simulink model "ModelMarco_Full"  (R2018a)
settings: Solver=FixedStepAuto  StartTime=0  StopTime=1382400  FixedStep=5  RelTol=1e-1
undefined symbols (not defined in the file or in its folder): magnitude
libraries: simulink x2
(part 2 of 2)

== system ModelMarco_Full/RoofStrategy ==
  Tset_vent : Inport
  RHset_vent : Inport  Port=2
  T_air : Inport  Port=3
  RH : Inport  Port=4
  RH_out : Inport  Port=5
  I : Inport  Port=6
  Constant : Constant  Value=0
  Gain : Gain
  Gain1 : Gain  Gain=0
  MATLAB Function : MATLAB Function  TreatAsAtomicUnit=on
  MATLAB Function1 : MATLAB Function  TreatAsAtomicUnit=on
  Saturation : Saturate  UpperLimit=1  LowerLimit=0
  Scope : Scope
  Sum : Sum  Inputs=|++
  day/night : Switch  Criteria=u2 > Threshold  Threshold=20
  Uroof : Outport
  wires:
  T_air/1 -> MATLAB Function/1(T_air)
  Tset_vent/1 -> MATLAB Function/2(Tset)
  RH/1 -> MATLAB Function1/1(RH_air)
  RH_out/1 -> MATLAB Function1/2(RH_out)
  RHset_vent/1 -> MATLAB Function1/3(RH_set)
  MATLAB Function/1(y) -> Gain/1
  MATLAB Function1/1(y) -> Gain1/1
  Gain/1 -> Sum/1
  Gain1/1 -> Sum/2
  Sum/1 -> Saturation/1
  I/1 -> day/night/2
  day/night/1 -> Scope/1, Uroof/1
  Saturation/1 -> day/night/1
  Constant/1 -> day/night/3

== system ModelMarco_Full/Scr(Scr->Covin) ==
  A_floor : Inport
  T_scr : Inport  Port=2
  T_covin : Inport  Port=3
  U_Thrscr : Inport  Port=4
  " Stefan-Boltzmann constant" : Constant  Value=5.67e-8
  " epsilon_cov" : Constant  Value=0.9
  " epsilon_scr" : Constant  Value=0.44
  Bias : Bias  Bias=273.15
  Bias1 : Bias  Bias=273.15
  Fcn : Fcn  Expr=u^4
  Fcn1 : Fcn  Expr=u^4
  Product : Product  Inputs=6
  Sum : Sum  Inputs=|+-
  R_FIR_scr->covin : Outport
  wires:
  A_floor/1 -> Product/1  "A_floor"
  T_scr/1 -> Bias/1
  T_covin/1 -> Bias1/1
  Bias/1 -> Fcn/1
  Bias1/1 -> Fcn1/1
  Fcn/1 -> Sum/1
  Fcn1/1 -> Sum/2
  Sum/1 -> Product/3
  Product/1 -> R_FIR_scr->covin/1
  " Stefan-Boltzmann constant"/1 -> Product/4
  " epsilon_cov"/1 -> Product/2
  U_Thrscr/1 -> Product/5  "F"
  " epsilon_scr"/1 -> Product/6

== system ModelMarco_Full/Scr(Scr->sky) ==
  A_floor : Inport
  T_scr : Inport  Port=2
  T_sky : Inport  Port=3
  U_Thrscr : Inport  Port=4
  " Stefan-Boltzmann constant" : Constant  Value=5.67e-8
  " epsilon_scr" : Constant  Value=0.44
  " epsilon_sky" : Constant
  Bias : Bias  Bias=273.15
  Bias1 : Bias  Bias=273.15
  Fcn : Fcn  Expr=u^4
  Fcn1 : Fcn  Expr=u^4
  Product : Product  Inputs=6
  Sum : Sum  Inputs=|+-
  tau_cov : Gain  Gain=0
  R_FIR_scr->sky : Outport
  wires:
  A_floor/1 -> Product/1  "A_floor"
  T_scr/1 -> Bias/1
  T_sky/1 -> Bias1/1
  Bias/1 -> Fcn/1
  Bias1/1 -> Fcn1/1
  Fcn/1 -> Sum/1
  Fcn1/1 -> Sum/2
  Sum/1 -> Product/3
  Product/1 -> R_FIR_scr->sky/1
  " Stefan-Boltzmann constant"/1 -> Product/4
  " epsilon_sky"/1 -> Product/2
  U_Thrscr/1 -> tau_cov/1
  tau_cov/1 -> Product/5  "F"
  " epsilon_scr"/1 -> Product/6

== system ModelMarco_Full/Scr(can->scr) ==
  A_floor : Inport
  T_can : Inport  Port=2
  T_scr : Inport  Port=3
  U_Thrscr : Inport  Port=4
  LAI : Inport  Port=5
  " Stefan-Boltzmann constant" : Constant  Value=5.67e-8
  " epsilon_can" : Constant
  " epsilon_scr" : Constant  Value=0.44
  Bias : Bias  Bias=273.15
  Bias1 : Bias  Bias=273.15
  Fcn : Fcn  Expr=u^4
  Fcn1 : Fcn  Expr=u^4
  Fcn2 : Fcn  Expr=1-exp(-0.94*u)
  Product : Product  Inputs=6
  Product1 : Product
  Sum : Sum  Inputs=|+-
  R_FIR_can->scr : Outport
  wires:
  T_can/1 -> Bias/1
  T_scr/1 -> Bias1/1
  Bias/1 -> Fcn/1
  Bias1/1 -> Fcn1/1
  Fcn/1 -> Sum/1
  Fcn1/1 -> Sum/2
  Sum/1 -> Product/3
  Product/1 -> R_FIR_can->scr/1
  " Stefan-Boltzmann constant"/1 -> Product/4
  " epsilon_scr"/1 -> Product/2
  U_Thrscr/1 -> Product/5  "F"
  " epsilon_can"/1 -> Product/6
  LAI/1 -> Fcn2/1
  Product1/1 -> Product/1
  A_floor/1 -> Product1/2  "A_floor"
  Fcn2/1 -> Product1/1

== system ModelMarco_Full/Scr(floor->scr) ==
  A_floor : Inport
  T_floor : Inport  Port=2
  T_scr : Inport  Port=3
  U_Thrscr : Inport  Port=4
  LAI : Inport  Port=5
  " Stefan-Boltzmann constant" : Constant  Value=5.67e-8
  " epsilon_floor" : Constant
  " epsilon_scr" : Constant  Value=0.44
  Bias : Bias  Bias=273.15
  Bias1 : Bias  Bias=273.15
  Fcn : Fcn  Expr=u^4
  Fcn1 : Fcn  Expr=u^4
  Fcn2 : Fcn  Expr=exp(-0.94*u)
  Product : Product  Inputs=6
  Product1 : Product
  Sum : Sum  Inputs=|+-
  R_FIR_floor->scr : Outport
  wires:
  T_floor/1 -> Bias/1
  T_scr/1 -> Bias1/1
  Bias/1 -> Fcn/1
  Bias1/1 -> Fcn1/1
  Fcn/1 -> Sum/1
  Fcn1/1 -> Sum/2
  Sum/1 -> Product/3
  Product/1 -> R_FIR_floor->scr/1
  " Stefan-Boltzmann constant"/1 -> Product/4
  " epsilon_scr"/1 -> Product/2
  " epsilon_floor"/1 -> Product/6
  A_floor/1 -> Product/1
  LAI/1 -> Fcn2/1
  Product1/1 -> Product/5
  Fcn2/1 -> Product1/1
  U_Thrscr/1 -> Product1/2

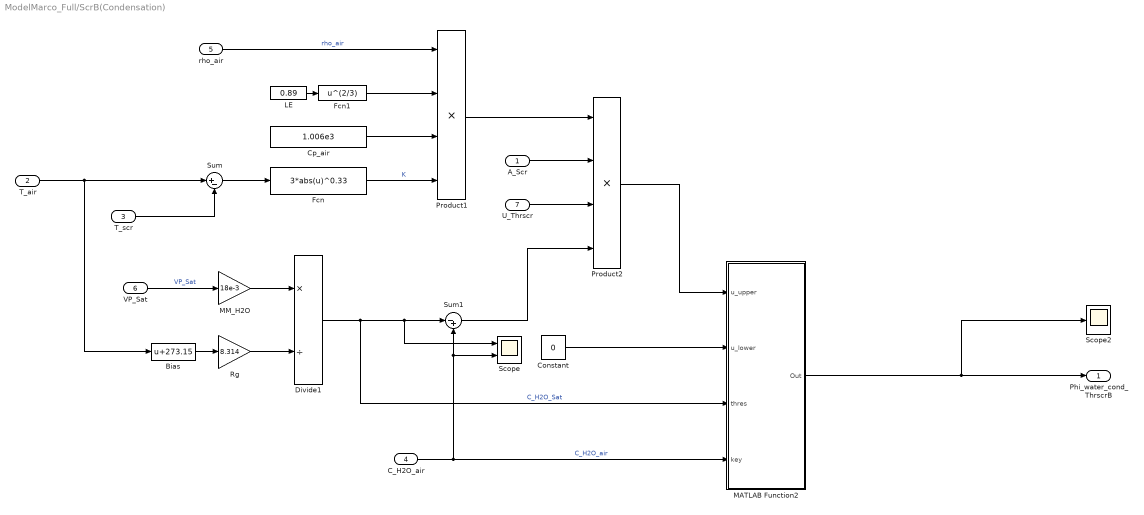
== system ModelMarco_Full/ScrB(Condensation) ==
  A_Scr : Inport
  T_air : Inport  Port=2
  T_scr : Inport  Port=3
  C_H2O_air : Inport  Port=4
  rho_air : Inport  Port=5
  VP_Sat : Inport  Port=6
  U_Thrscr : Inport  Port=7
  Bias : Bias  Bias=273.15
  Constant : Constant  Value=0
  Cp_air : Constant  Value=1.006e3
  Divide1 : Product  Inputs=*/
  Fcn : Fcn  Expr=3*abs(u)^0.33
  Fcn1 : Fcn  Expr=u^(2/3)
  LE : Constant  Value=0.89
  MATLAB Function2 : MATLAB Function  TreatAsAtomicUnit=on
  MM_H2O : Gain  Gain=18e-3
  Product1 : Product  Inputs=4
  Product2 : Product  Inputs=4
  Rg : Gain  Gain=8.314
  Scope : Scope  NumInputPorts=2
  Scope2 : Scope
  Sum : Sum  Inputs=|+-
  Sum1 : Sum  Inputs=|-+
  Phi_water_cond_ThrscrB : Outport
  wires:
  T_air/1 -> Sum/1, Bias/1
  T_scr/1 -> Sum/2
  Sum/1 -> Fcn/1
  Bias/1 -> Rg/1
  Rg/1 -> Divide1/2
  rho_air/1 -> Product1/1  "rho_air"
  LE/1 -> Fcn1/1
  Fcn1/1 -> Product1/2
  Cp_air/1 -> Product1/3
  Fcn/1 -> Product1/4  "K"
  VP_Sat/1 -> MM_H2O/1  "VP_Sat"
  MM_H2O/1 -> Divide1/1
  Divide1/1 -> MATLAB Function2/3(thres), Scope/1, Sum1/1  "C_H2O_Sat"
  C_H2O_air/1 -> Scope/2, Sum1/2, MATLAB Function2/4(key)  "C_H2O_air"
  Product1/1 -> Product2/1
  A_Scr/1 -> Product2/2
  Constant/1 -> MATLAB Function2/2(u_lower)
  Product2/1 -> MATLAB Function2/1(u_upper)
  MATLAB Function2/1(Out) -> Scope2/1, Phi_water_cond_ThrscrB/1
  Sum1/1 -> Product2/4
  U_Thrscr/1 -> Product2/3

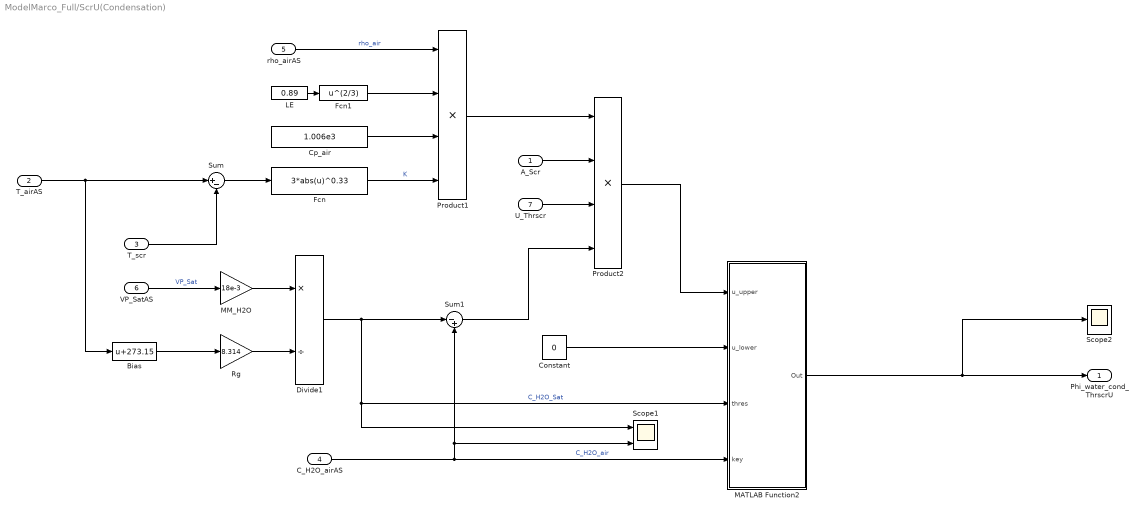
== system ModelMarco_Full/ScrU(Condensation) ==
  A_Scr : Inport
  T_airAS : Inport  Port=2
  T_scr : Inport  Port=3
  C_H2O_airAS : Inport  Port=4
  rho_airAS : Inport  Port=5
  VP_SatAS : Inport  Port=6
  U_Thrscr : Inport  Port=7
  Bias : Bias  Bias=273.15
  Constant : Constant  Value=0
  Cp_air : Constant  Value=1.006e3
  Divide1 : Product  Inputs=*/
  Fcn : Fcn  Expr=3*abs(u)^0.33
  Fcn1 : Fcn  Expr=u^(2/3)
  LE : Constant  Value=0.89
  MATLAB Function2 : MATLAB Function  TreatAsAtomicUnit=on
  MM_H2O : Gain  Gain=18e-3
  Product1 : Product  Inputs=4
  Product2 : Product  Inputs=4
  Rg : Gain  Gain=8.314
  Scope1 : Scope  NumInputPorts=2
  Scope2 : Scope
  Sum : Sum  Inputs=|+-
  Sum1 : Sum  Inputs=|-+
  Phi_water_cond_ThrscrU : Outport
  wires:
  T_airAS/1 -> Sum/1, Bias/1
  T_scr/1 -> Sum/2
  Sum/1 -> Fcn/1
  Bias/1 -> Rg/1
  Rg/1 -> Divide1/2
  rho_airAS/1 -> Product1/1  "rho_air"
  LE/1 -> Fcn1/1
  Fcn1/1 -> Product1/2
  Cp_air/1 -> Product1/3
  Fcn/1 -> Product1/4  "K"
  VP_SatAS/1 -> MM_H2O/1  "VP_Sat"
  MM_H2O/1 -> Divide1/1
  Divide1/1 -> Scope1/1, MATLAB Function2/3(thres), Sum1/1  "C_H2O_Sat"
  C_H2O_airAS/1 -> Scope1/2, Sum1/2, MATLAB Function2/4(key)  "C_H2O_air"
  Product1/1 -> Product2/1
  A_Scr/1 -> Product2/2
  Constant/1 -> MATLAB Function2/2(u_lower)
  Product2/1 -> MATLAB Function2/1(u_upper)
  MATLAB Function2/1(Out) -> Scope2/1, Phi_water_cond_ThrscrU/1
  Sum1/1 -> Product2/4
  U_Thrscr/1 -> Product2/3

== system ModelMarco_Full/Screen(Air->airAS) ==
  Phi_airASair : Inport
  T_air : Inport  Port=2
  T_airAS : Inport  Port=3
  Cp_air : Constant  Value=1.006e3
  Product : Product  Inputs=3
  Sum : Sum  Inputs=|+-
  Q_air->airAS : Outport
  wires:
  T_air/1 -> Sum/1
  T_airAS/1 -> Sum/2
  Sum/1 -> Product/3
  Cp_air/1 -> Product/1
  Phi_airASair/1 -> Product/2
  Product/1 -> Q_air->airAS/1

== system ModelMarco_Full/Screen(AirAs->scr) ==
  A_floor : Inport
  T_scr : Inport  Port=2
  T_airAS : Inport  Port=3
  U_Thrscr : Inport  Port=4
  Fcn : Fcn  Expr=1.7*abs(u)^0.33
  Product : Product  Inputs=3
  Product1 : Product
  Sum : Sum  Inputs=|+-
  Q_airAS->scr : Outport
  wires:
  T_airAS/1 -> Sum/1
  T_scr/1 -> Sum/2
  Sum/1 -> Fcn/1, Product/2
  A_floor/1 -> Product/1
  Product1/1 -> Product/3  "K"
  Fcn/1 -> Product1/1
  U_Thrscr/1 -> Product1/2
  Product/1 -> Q_airAS->scr/1

== system ModelMarco_Full/Screen(scr->air) ==
  A_floor : Inport
  T_air : Inport  Port=2
  T_scr : Inport  Port=3
  U_Thrscr : Inport  Port=4
  Fcn : Fcn  Expr=1.7*abs(u)^0.33
  Product : Product  Inputs=3
  Product1 : Product
  Sum : Sum  Inputs=|+-
  Q_scrair : Outport
  wires:
  T_scr/1 -> Sum/1
  T_air/1 -> Sum/2
  Sum/1 -> Fcn/1, Product/2
  A_floor/1 -> Product/1
  Product1/1 -> Product/3  "K"
  Fcn/1 -> Product1/1
  U_Thrscr/1 -> Product1/2
  Product/1 -> Q_scrair/1

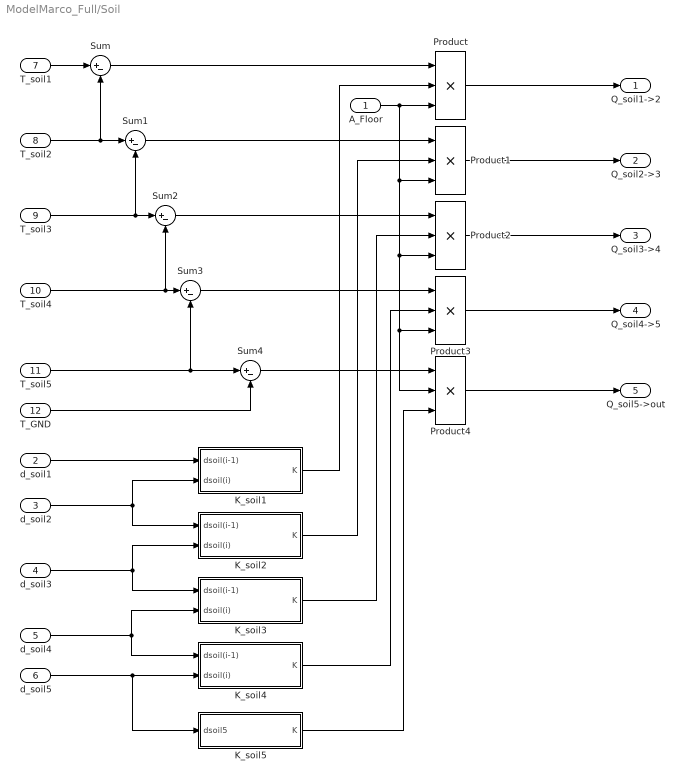
== system ModelMarco_Full/Soil ==
  A_Floor : Inport
  d_soil1 : Inport  Port=2
  d_soil2 : Inport  Port=3
  d_soil3 : Inport  Port=4
  d_soil4 : Inport  Port=5
  d_soil5 : Inport  Port=6
  T_soil1 : Inport  Port=7
  T_soil2 : Inport  Port=8
  T_soil3 : Inport  Port=9
  T_soil4 : Inport  Port=10
  T_soil5 : Inport  Port=11
  T_GND : Inport  Port=12
  K_soil1 : Subsystem
  K_soil2 : Subsystem
  K_soil3 : Subsystem
  K_soil4 : Subsystem
  K_soil5 : Subsystem
  Product{,1..4} (5 alike) : Product  Inputs=3
  Sum{,1..4} (5 alike) : Sum  Inputs=|+-
  Q_soil1->2 : Outport
  Q_soil2->3 : Outport  Port=2
  Q_soil3->4 : Outport  Port=3
  Q_soil4->5 : Outport  Port=4
  Q_soil5->out : Outport  Port=5
  wires:
  d_soil2/1 -> K_soil1/2(dsoil(i)), K_soil2/1(dsoil(i-1))
  d_soil1/1 -> K_soil1/1(dsoil(i-1))
  d_soil3/1 -> K_soil3/1(dsoil(i-1)), K_soil2/2(dsoil(i))
  d_soil4/1 -> K_soil3/2(dsoil(i)), K_soil4/1(dsoil(i-1))
  d_soil5/1 -> K_soil5/1(dsoil5), K_soil4/2(dsoil(i))
  T_soil1/1 -> Sum/1
  T_soil2/1 -> Sum/2, Sum1/1
  Sum/1 -> Product/1
  K_soil1/1(K) -> Product/2
  A_Floor/1 -> Product2/3, Product4/2, Product3/3, Product1/3, Product/3
  Product/1 -> Q_soil1->2/1
  Sum1/1 -> Product1/1
  K_soil2/1(K) -> Product1/2
  Product1/1 -> Q_soil2->3/1
  T_soil3/1 -> Sum2/1, Sum1/2
  Sum2/1 -> Product2/1
  T_soil4/1 -> Sum3/1, Sum2/2
  Sum3/1 -> Product3/1
  K_soil3/1(K) -> Product2/2
  T_soil5/1 -> Sum3/2, Sum4/1
  K_soil4/1(K) -> Product3/2
  Product2/1 -> Q_soil3->4/1
  Product3/1 -> Q_soil4->5/1
  T_GND/1 -> Sum4/2
  Sum4/1 -> Product4/1
  K_soil5/1(K) -> Product4/3
  Product4/1 -> Q_soil5->out/1

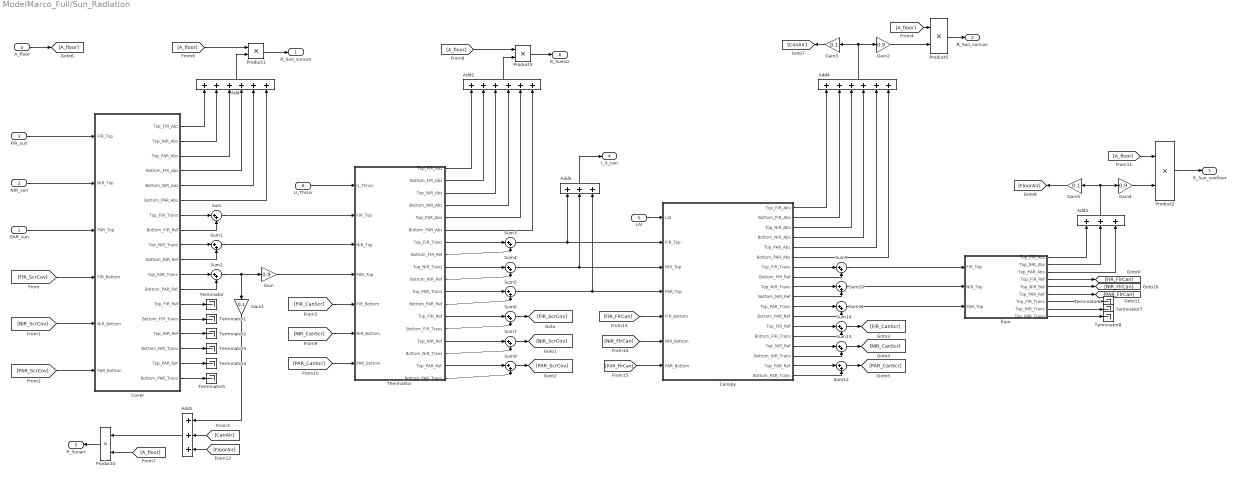
== system ModelMarco_Full/Sun_Radiation ==
  PAR_sun : Inport
  NIR_sun : Inport  Port=2
  FIR_sun : Inport  Port=3
  A_floor : Inport  Port=4
  LAI : Inport  Port=5
  U_Thrscr : Inport  Port=6
  Add : Sum  Inputs=++++++
  Add1 : Sum  Inputs=+++
  Add2 : Sum  Inputs=++++++
  Add3 : Sum  Inputs=+++
  Add4 : Sum  Inputs=++++++
  Add5 : Sum  Inputs=+++
  Canopy : Subsystem
  Cover : Subsystem
  Gain : Gain  Gain=0.9
  Gain1 : Gain  Gain=0.1
  Gain2 : Gain  Gain=0.9
  Gain3 : Gain  Gain=0.1
  Gain4 : Gain  Gain=0.9
  Gain5 : Gain  Gain=0.1
  Product{1..5} (5 alike) : Product
  Sum{,1..14} (15 alike) : Sum  Inputs=|++
  Terminator{,1..8} (9 alike) : Terminator
  ThermalScr : Subsystem
  floor : Subsystem
  R_Sun_suncov : Outport
  R_Sun_suncan : Outport  Port=2
  R_Sun_sunfloor : Outport  Port=3
  I_A_can : Outport  Port=4
  R_Sunair : Outport  Port=5
  "R_Sunscr " : Outport  Port=6
  wires:
  [FIR_ScrCov] -> Cover/4(FIR_Bottom)
  [NIR_ScrCov] -> Cover/5(NIR_Bottom)
  [PAR_ScrCov] -> Cover/6(PAR_Bottom)
  Product2/1 -> R_Sun_sunfloor/1
  [FIR_FlrCan] -> Canopy/5(FIR_Bottom)
  [NIR_FlrCan] -> Canopy/6(NIR_Bottom)
  [PAR_FlrCan] -> Canopy/7(PAR_Bottom)
  PAR_sun/1 -> Cover/3(PAR_Top)
  A_floor/1 -> [A_floor]
  LAI/1 -> Canopy/1(LAI)
  Cover/1(Top_FIR_Abs) -> Add/1
  Cover/2(Top_NIR_Abs) -> Add/2
  Cover/3(Top_PAR_Abs) -> Add/3
  Cover/4(Bottom_FIR_Abs) -> Add/4
  Cover/5(Bottom_NIR_Abs) -> Add/5
  Cover/6(Bottom_PAR_Abs) -> Add/6
  [A_floor] -> Product1/1
  Add/1 -> Product1/2
  Product1/1 -> R_Sun_suncov/1
  Cover/7(Top_FIR_Trans) -> Sum/1
  Cover/8(Bottom_FIR_Ref) -> Sum/2
  Cover/9(Top_NIR_Trans) -> Sum1/1
  Cover/10(Bottom_NIR_Ref) -> Sum1/2
  Cover/11(Top_PAR_Trans) -> Sum2/1
  Cover/12(Bottom_PAR_Ref) -> Sum2/2
  Sum/1 -> ThermalScr/2(FIR_Top)
  Sum1/1 -> ThermalScr/3(NIR_Top)
  Cover/13(Top_FIR_Ref) -> Terminator/1
  Cover/14(Bottom_FIR_Trans) -> Terminator1/1
  Cover/15(Top_NIR_Ref) -> Terminator2/1
  Cover/16(Bottom_NIR_Trans) -> Terminator3/1
  Cover/17(Top_PAR_Ref) -> Terminator4/1
  Cover/18(Bottom_PAR_Trans) -> Terminator5/1
  U_Thrscr/1 -> ThermalScr/1(U_Thrscr)
  NIR_sun/1 -> Cover/2(NIR_Top)
  FIR_sun/1 -> Cover/1(FIR_Top)
  Gain/1 -> ThermalScr/4(PAR_Top)
  Sum2/1 -> Gain1/1, Gain/1
  Gain1/1 -> Add1/1
  Add1/1 -> Product4/1
  [A_floor] -> Product4/2
  Product4/1 -> R_Sunair/1
  ThermalScr/1(Top_FIR_Abs) -> Add2/1
  ThermalScr/2(Bottom_FIR_Abs) -> Add2/2
  ThermalScr/3(Top_NIR_Abs) -> Add2/3
  ThermalScr/4(Bottom_NIR_Abs) -> Add2/4
  ThermalScr/5(Top_PAR_Abs) -> Add2/5
  ThermalScr/6(Bottom_PAR_Abs) -> Add2/6
  [A_floor] -> Product3/1
  Add2/1 -> Product3/2
  Product3/1 -> "R_Sunscr "/1
  ThermalScr/7(Top_FIR_Trans) -> Sum3/1
  ThermalScr/8(Bottom_FIR_Ref) -> Sum3/2
  ThermalScr/9(Top_NIR_Trans) -> Sum4/1
  ThermalScr/10(Bottom_NIR_Ref) -> Sum4/2
  ThermalScr/11(Top_PAR_Trans) -> Sum5/1
  ThermalScr/12(Bottom_PAR_Ref) -> Sum5/2
  Sum3/1 -> Add5/1, Canopy/2(FIR_Top)
  Sum4/1 -> Add5/2, Canopy/3(NIR_Top)
  Sum5/1 -> Add5/3, Canopy/4(PAR_Top)
  Sum6/1 -> [FIR_ScrCov]
  ThermalScr/13(Top_FIR_Ref) -> Sum6/1
  ThermalScr/14(Bottom_FIR_Trans) -> Sum6/2
  ThermalScr/15(Top_NIR_Ref) -> Sum7/1
  ThermalScr/16(Bottom_NIR_Trans) -> Sum7/2
  Sum7/1 -> [NIR_ScrCov]
  ThermalScr/17(Top_PAR_Ref) -> Sum8/1
  ThermalScr/18(Bottom_PAR_Trans) -> Sum8/2
  Sum8/1 -> [PAR_ScrCov]
  Canopy/1(Top_FIR_Abs) -> Add4/1
  Canopy/2(Bottom_FIR_Abs) -> Add4/2
  Canopy/3(Top_NIR_Abs) -> Add4/3
  Canopy/4(Bottom_NIR_Abs) -> Add4/4
  Canopy/5(Top_PAR_Abs) -> Add4/5
  Canopy/6(Bottom_PAR_Abs) -> Add4/6
  Add4/1 -> Gain2/1, Gain3/1
  Gain3/1 -> [CanAir]
  [CanAir] -> Add1/2
  Product5/1 -> R_Sun_suncan/1
  [A_floor] -> Product5/1
  Gain2/1 -> Product5/2
  Canopy/7(Top_FIR_Trans) -> Sum9/1
  Canopy/9(Top_NIR_Trans) -> Sum10/1
  Canopy/11(Top_PAR_Trans) -> Sum11/1
  Canopy/8(Bottom_FIR_Ref) -> Sum9/2
  Canopy/10(Bottom_NIR_Ref) -> Sum10/2
  Canopy/12(Bottom_PAR_Ref) -> Sum11/2
  Sum9/1 -> floor/1(FIR_Top)
  Sum10/1 -> floor/2(NIR_Top)
  Sum11/1 -> floor/3(PAR_Top)
  Canopy/13(Top_FIR_Ref) -> Sum14/1
  Canopy/14(Bottom_FIR_Trans) -> Sum14/2
  Canopy/15(Top_NIR_Ref) -> Sum13/1
  Canopy/16(Bottom_NIR_Trans) -> Sum13/2
  Canopy/17(Top_PAR_Ref) -> Sum12/1
  Canopy/18(Bottom_PAR_Trans) -> Sum12/2
  Add5/1 -> I_A_can/1
  Sum14/1 -> [FIR_CanScr]
  Sum13/1 -> [NIR_CanScr]
  Sum12/1 -> [PAR_CanScr]
  [FIR_CanScr] -> ThermalScr/5(FIR_Bottom)
  [NIR_CanScr] -> ThermalScr/6(NIR_Bottom)
  [PAR_CanScr] -> ThermalScr/7(PAR_Bottom)
  floor/1(Top_FIR_Abs) -> Add3/1
  floor/2(Top_NIR_Abs) -> Add3/2
  floor/3(Top_PAR_Abs) -> Add3/3
  Add3/1 -> Gain4/1, Gain5/1
  Gain4/1 -> Product2/2
  [A_floor] -> Product2/1
  Gain5/1 -> [FloorAir]
  [FloorAir] -> Add1/3
  floor/9(Top_PAR_Trans) -> Terminator8/1
  floor/8(Top_NIR_Trans) -> Terminator7/1
  floor/7(Top_FIR_Trans) -> Terminator6/1
  floor/4(Top_FIR_Ref) -> [FIR_FlrCan]
  floor/5(Top_NIR_Ref) -> [NIR_FlrCan]
  floor/6(Top_PAR_Ref) -> [PAR_FlrCan]

== system ModelMarco_Full/Vent ==
  rho_airAS : Inport
  Phi_roofvent : Inport  Port=2
  T_airAS : Inport  Port=3
  Tout : Inport  Port=4
  Cp_air : Constant  Value=1.006e3
  Product : Product  Inputs=4
  Sum : Sum  Inputs=|+-
  Q_roofvent : Outport
  wires:
  T_airAS/1 -> Sum/1
  Tout/1 -> Sum/2
  Sum/1 -> Product/4
  rho_airAS/1 -> Product/2
  Phi_roofvent/1 -> Product/3
  Cp_air/1 -> Product/1
  Product/1 -> Q_roofvent/1

== system ModelMarco_Full/Wall(air->out) ==
  Tout : Inport
  Tair : Inport  Port=2
  U : Inport  Port=3
  A_wall : Inport  Port=4
  Gain : Gain
  Product : Product  Inputs=3
  Sum : Sum  Inputs=|+-
  Q_air->out : Outport
  wires:
  Tair/1 -> Sum/1
  Tout/1 -> Sum/2
  Sum/1 -> Product/3
  U/1 -> Product/2
  A_wall/1 -> Product/1
  Gain/1 -> Q_air->out/1
  Product/1 -> Gain/1

== system ModelMarco_Full/Water_flow(ThrScr) ==
  Phi_leakage : Inport
  C_H2O_Air : Inport  Port=2
  C_H2O_AirAs : Inport  Port=3
  Product : Product
  Sum : Sum  Inputs=|+-
  Phi_water_ThrScr : Outport
  wires:
  C_H2O_Air/1 -> Sum/1
  C_H2O_AirAs/1 -> Sum/2
  Phi_leakage/1 -> Product/1
  Sum/1 -> Product/2
  Product/1 -> Phi_water_ThrScr/1

== system ModelMarco_Full/Water_flow(leakage) ==
  Phi_leakage : Inport
  C_H2O_in : Inport  Port=2
  C_H2O_out : Inport  Port=3
  Product : Product
  Sum : Sum  Inputs=|+-
  Phi_water_leak : Outport
  wires:
  C_H2O_in/1 -> Sum/1
  C_H2O_out/1 -> Sum/2
  Phi_leakage/1 -> Product/1
  Sum/1 -> Product/2
  Product/1 -> Phi_water_leak/1

== system ModelMarco_Full/Water_flow(roofvent) ==
  Phi_roofvent : Inport
  C_H2O_AS : Inport  Port=2
  C_H2O_out : Inport  Port=3
  Product : Product
  Sum : Sum  Inputs=|+-
  Phi_water_roofvent : Outport
  wires:
  C_H2O_AS/1 -> Sum/1
  C_H2O_out/1 -> Sum/2
  Phi_roofvent/1 -> Product/1
  Sum/1 -> Product/2
  Product/1 -> Phi_water_roofvent/1

== system ModelMarco_Full/Plants(transpiration)/Boundary Resistance ==
  note: Different Paper give different suggestion, not senstive
  T_can : Inport
  T_air : Inport  Port=2
  Abs : Abs
  Divide1 : Product  Inputs=**/
  Fcn : Fcn  Expr=u^(2/3)
  Fcn1 : Fcn  Expr=u^(1/4)
  Gain : Gain  Gain=1147
  Gain1 : Gain  Gain=207
  Le : Constant  Value=0.89
  Lf : Constant  Value=0.055
  Manual Switch : ManualSwitch  CurrentSetting=0
  Math Function : Math  Operator=magnitude^2  SaturateOnIntegerOverflow=on
  Product2 : Product
  Sqrt : Sqrt  SaturateOnIntegerOverflow=on
  Sum : Sum  Inputs=|+-
  Sum1 : Sum  Inputs=|++
  Vair : Constant  Value=0.08
  rb : Constant  Value=100
  r_b : Outport
  wires:
  Math Function/1 -> Gain1/1
  Sqrt/1 -> Gain/1
  Vair/1 -> Math Function/1
  Fcn/1 -> Divide1/1
  Divide1/1 -> Manual Switch/1  "r_b"
  Abs/1 -> Product2/2
  Sum1/1 -> Fcn1/1
  Gain1/1 -> Sum1/2
  T_air/1 -> Sum/2
  Sum/1 -> Abs/1
  Product2/1 -> Sum1/1
  Lf/1 -> Sqrt/1, Product2/1
  Gain/1 -> Divide1/2
  Fcn1/1 -> Divide1/3
  Le/1 -> Fcn/1
  rb/1 -> Manual Switch/2
  T_can/1 -> Sum/1
  Manual Switch/1 -> r_b/1

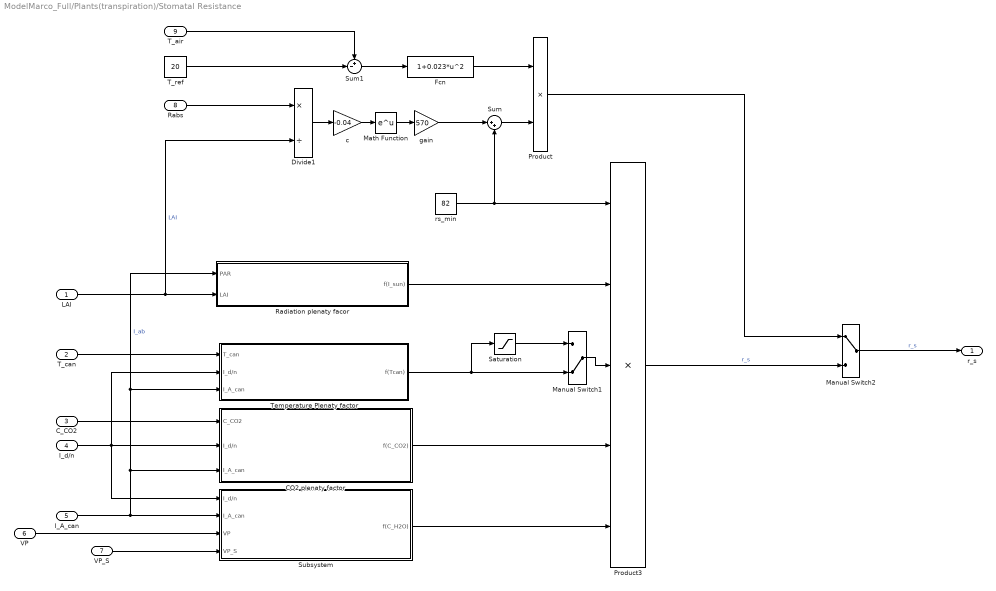
== system ModelMarco_Full/Plants(transpiration)/Stomatal Resistance  ==
  LAI : Inport
  T_can : Inport  Port=2
  C_CO2 : Inport  Port=3
  I_d/n : Inport  Port=4
  I_A_can : Inport  Port=5
  VP : Inport  Port=6
  VP_S : Inport  Port=7
  Rabs : Inport  Port=8
  T_air : Inport  Port=9
  CO2 plenaty factor : Subsystem
  Divide1 : Product  Inputs=*/
  Fcn : Fcn  Expr=1+0.023*u^2
  Manual Switch1 : ManualSwitch  CurrentSetting=0
  Manual Switch2 : ManualSwitch
  Math Function : Math  SaturateOnIntegerOverflow=on
  Product : Product
  Product3 : Product  Inputs=5
  Radiation plenaty facor : Subsystem
  Saturation : Saturate  UpperLimit=1
  Subsystem : Subsystem
  Sum : Sum  Inputs=|++
  Sum1 : Sum  Inputs=+-|
  T_ref : Constant  Value=20
  Temperature Plenaty factor : Subsystem
  c : Gain  Gain=-0.04
  gain : Gain  Gain=570
  rs_min : Constant  Value=82
  r_s : Outport
  wires:
  Manual Switch1/1 -> Product3/3
  CO2 plenaty factor/1(f(C_CO2)) -> Product3/4
  Subsystem/1(f(C_H2O)) -> Product3/5
  Radiation plenaty facor/1(f(I_sun)) -> Product3/2
  I_d/n/1 -> Subsystem/1(I_d/n), CO2 plenaty factor/2(I_d/n), Temperature Plenaty factor/2(I_d/n)
  rs_min/1 -> Sum/2, Product3/1
  Temperature Plenaty factor/1(f(Tcan)) -> Saturation/1, Manual Switch1/2
  C_CO2/1 -> CO2 plenaty factor/1(C_CO2)
  VP/1 -> Subsystem/3(VP)
  LAI/1 -> Divide1/2, Radiation plenaty facor/2(LAI)  "LAI"
  T_can/1 -> Temperature Plenaty factor/1(T_can)
  VP_S/1 -> Subsystem/4(VP_S)
  Saturation/1 -> Manual Switch1/1
  Manual Switch2/1 -> r_s/1  "r_s"
  Product3/1 -> Manual Switch2/2  "r_s"
  I_A_can/1 -> Radiation plenaty facor/1(PAR), Temperature Plenaty factor/3(I_A_can), CO2 plenaty factor/3(I_A_can), Subsystem/2(I_A_can)  "I_ab"
  Divide1/1 -> c/1
  c/1 -> Math Function/1
  Math Function/1 -> gain/1
  Rabs/1 -> Divide1/1
  gain/1 -> Sum/1
  Sum/1 -> Product/2
  Fcn/1 -> Product/1
  Product/1 -> Manual Switch2/1
  T_ref/1 -> Sum1/2
  T_air/1 -> Sum1/1
  Sum1/1 -> Fcn/1

== system ModelMarco_Full/Plants(transpiration)/Vapour Pressure Air ==
  C_H2O : Inport
  VP_sat : Inport  Port=2
  T_air : Inport  Port=3
  Divide4 : Product  Inputs=*/
  Divide5 : Product  Inputs=**/
  Fcn3 : Fcn  Expr=8.314*(u+273.15)
  Gain7 : Gain  Gain=18e-3
  VP : Outport
  wires:
  Gain7/1 -> Divide4/1
  Divide4/1 -> Divide5/3  "C_H2O_sat"
  VP_sat/1 -> Gain7/1, Divide5/2
  C_H2O/1 -> Divide5/1
  Fcn3/1 -> Divide4/2
  T_air/1 -> Fcn3/1
  Divide5/1 -> VP/1  "VP"

== system ModelMarco_Full/Plants(transpiration)/vapour transfer coefficient  ==
  rho_air : Inport
  R : Inport  Port=2
  Cp_air : Constant  Value=1.006e3
  Divide : Product  Inputs=**/
  LH : Constant  Value=2.45e6
  Product1 : Product  Inputs=3
  gamma : Constant  Value=65.8
  K : Outport
  wires:
  Cp_air/1 -> Divide/2
  gamma/1 -> Product1/2
  Product1/1 -> Divide/3
  R/1 -> Product1/3
  LH/1 -> Product1/1
  Divide/1 -> K/1  "K"
  rho_air/1 -> Divide/1

== system ModelMarco_Full/Soil/K_soil1 ==
  dsoil(i-1) : Inport
  dsoil(i) : Inport  Port=2
  Constant : Constant  Value=2
  Divide : Product  Inputs=*/
  Divide1 : Product  Inputs=*/
  Divide2 : Product  Inputs=*/
  Sum : Sum  Inputs=|++
  lambda_soil : Constant  Value=0.85
  K : Outport
  wires:
  dsoil(i-1)/1 -> Divide/1
  lambda_soil/1 -> Divide1/2, Divide/2
  dsoil(i)/1 -> Divide1/1
  Divide/1 -> Sum/1
  Divide1/1 -> Sum/2
  Sum/1 -> Divide2/2
  Constant/1 -> Divide2/1
  Divide2/1 -> K/1

== system ModelMarco_Full/Soil/K_soil2 ==
  dsoil(i-1) : Inport
  dsoil(i) : Inport  Port=2
  Constant : Constant  Value=2
  Divide : Product  Inputs=*/
  Divide1 : Product  Inputs=*/
  Divide2 : Product  Inputs=*/
  Sum : Sum  Inputs=|++
  lambda_soil : Constant  Value=0.85
  K : Outport
  wires:
  dsoil(i-1)/1 -> Divide/1
  lambda_soil/1 -> Divide1/2, Divide/2
  dsoil(i)/1 -> Divide1/1
  Divide/1 -> Sum/1
  Divide1/1 -> Sum/2
  Sum/1 -> Divide2/2
  Constant/1 -> Divide2/1
  Divide2/1 -> K/1

== system ModelMarco_Full/Soil/K_soil3 ==
  dsoil(i-1) : Inport
  dsoil(i) : Inport  Port=2
  Constant : Constant  Value=2
  Divide : Product  Inputs=*/
  Divide1 : Product  Inputs=*/
  Divide2 : Product  Inputs=*/
  Sum : Sum  Inputs=|++
  lambda_soil : Constant  Value=0.85
  K : Outport
  wires:
  dsoil(i-1)/1 -> Divide/1
  lambda_soil/1 -> Divide1/2, Divide/2
  dsoil(i)/1 -> Divide1/1
  Divide/1 -> Sum/1
  Divide1/1 -> Sum/2
  Sum/1 -> Divide2/2
  Constant/1 -> Divide2/1
  Divide2/1 -> K/1

== system ModelMarco_Full/Soil/K_soil4 ==
  dsoil(i-1) : Inport
  dsoil(i) : Inport  Port=2
  Constant : Constant  Value=2
  Divide : Product  Inputs=*/
  Divide1 : Product  Inputs=*/
  Divide2 : Product  Inputs=*/
  Sum : Sum  Inputs=|++
  lambda_soil : Constant  Value=0.85
  K : Outport
  wires:
  dsoil(i-1)/1 -> Divide/1
  lambda_soil/1 -> Divide1/2, Divide/2
  dsoil(i)/1 -> Divide1/1
  Divide/1 -> Sum/1
  Divide1/1 -> Sum/2
  Sum/1 -> Divide2/2
  Constant/1 -> Divide2/1
  Divide2/1 -> K/1

== system ModelMarco_Full/Soil/K_soil5 ==
  dsoil5 : Inport
  Constant : Constant
  Divide : Product  Inputs=*/
  Divide2 : Product  Inputs=*/
  lambda_soil : Constant  Value=0.85
  K : Outport
  wires:
  dsoil5/1 -> Divide/1
  lambda_soil/1 -> Divide/2
  Divide/1 -> Divide2/2
  Constant/1 -> Divide2/1
  Divide2/1 -> K/1

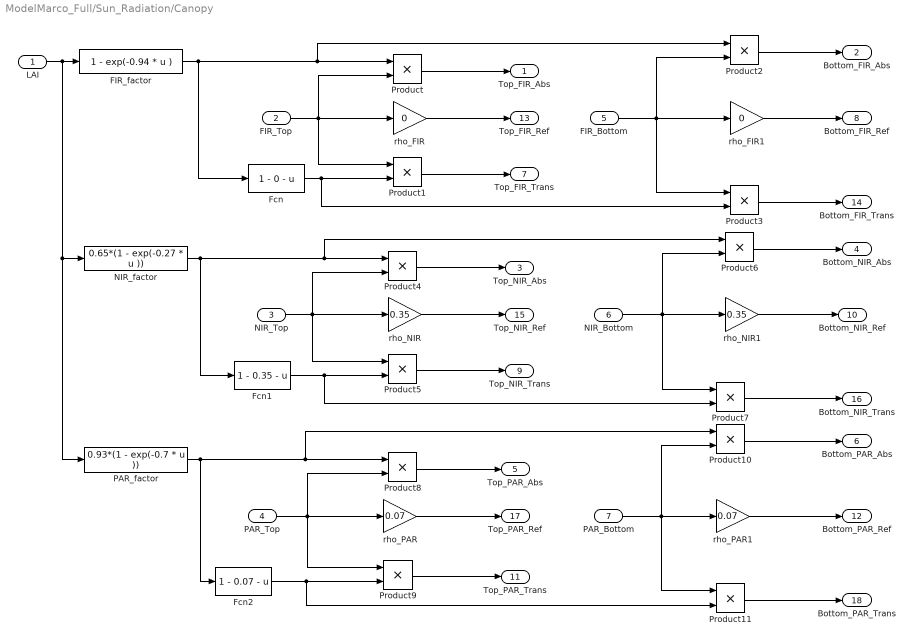
== system ModelMarco_Full/Sun_Radiation/Canopy ==
  LAI : Inport
  FIR_Top : Inport  Port=2
  NIR_Top : Inport  Port=3
  PAR_Top : Inport  Port=4
  FIR_Bottom : Inport  Port=5
  NIR_Bottom : Inport  Port=6
  PAR_Bottom : Inport  Port=7
  FIR_factor : Fcn  Expr=1 - exp(-0.94 * u )
  Fcn : Fcn  Expr=1 - 0 - u
  Fcn1 : Fcn  Expr=1 - 0.35 - u
  Fcn2 : Fcn  Expr=1 - 0.07 - u
  NIR_factor : Fcn  Expr=0.65*(1 - exp(-0.27 * u ))
  PAR_factor : Fcn  Expr=0.93*(1 - exp(-0.7 * u ))
  Product{,1..11} (12 alike) : Product
  rho_FIR : Gain  Gain=0
  rho_FIR1 : Gain  Gain=0
  rho_NIR : Gain  Gain=0.35
  rho_NIR1 : Gain  Gain=0.35
  rho_PAR : Gain  Gain=0.07
  rho_PAR1 : Gain  Gain=0.07
  Top_FIR_Abs : Outport
  Bottom_FIR_Abs : Outport  Port=2
  Top_NIR_Abs : Outport  Port=3
  Bottom_NIR_Abs : Outport  Port=4
  Top_PAR_Abs : Outport  Port=5
  Bottom_PAR_Abs : Outport  Port=6
  Top_FIR_Trans : Outport  Port=7
  Bottom_FIR_Ref : Outport  Port=8
  Top_NIR_Trans : Outport  Port=9
  Bottom_NIR_Ref : Outport  Port=10
  Top_PAR_Trans : Outport  Port=11
  Bottom_PAR_Ref : Outport  Port=12
  Top_FIR_Ref : Outport  Port=13
  Bottom_FIR_Trans : Outport  Port=14
  Top_NIR_Ref : Outport  Port=15
  Bottom_NIR_Trans : Outport  Port=16
  Top_PAR_Ref : Outport  Port=17
  Bottom_PAR_Trans : Outport  Port=18
  wires:
  Product1/1 -> Top_FIR_Trans/1
  rho_FIR/1 -> Top_FIR_Ref/1
  FIR_Top/1 -> Product1/1, Product/2, rho_FIR/1
  Product/1 -> Top_FIR_Abs/1
  FIR_Bottom/1 -> Product3/1, Product2/2, rho_FIR1/1
  rho_FIR1/1 -> Bottom_FIR_Ref/1
  Product2/1 -> Bottom_FIR_Abs/1
  rho_NIR/1 -> Top_NIR_Ref/1
  Product5/1 -> Top_NIR_Trans/1
  NIR_Top/1 -> rho_NIR/1, Product4/2, Product5/1
  Product4/1 -> Top_NIR_Abs/1
  rho_NIR1/1 -> Bottom_NIR_Ref/1
  NIR_Bottom/1 -> Product7/1, Product6/2, rho_NIR1/1
  Product6/1 -> Bottom_NIR_Abs/1
  Product7/1 -> Bottom_NIR_Trans/1
  PAR_Top/1 -> Product9/1, Product8/2, rho_PAR/1
  rho_PAR/1 -> Top_PAR_Ref/1
  Product8/1 -> Top_PAR_Abs/1
  Product11/1 -> Bottom_PAR_Trans/1
  rho_PAR1/1 -> Bottom_PAR_Ref/1
  Product10/1 -> Bottom_PAR_Abs/1
  PAR_Bottom/1 -> Product11/1, Product10/2, rho_PAR1/1
  LAI/1 -> PAR_factor/1, NIR_factor/1, FIR_factor/1
  FIR_factor/1 -> Fcn/1, Product2/1, Product/1
  Fcn/1 -> Product3/2, Product1/2
  Product3/1 -> Bottom_FIR_Trans/1
  NIR_factor/1 -> Fcn1/1, Product4/1, Product6/1
  Fcn1/1 -> Product5/2, Product7/2
  PAR_factor/1 -> Fcn2/1, Product10/1, Product8/1
  Product9/1 -> Top_PAR_Trans/1
  Fcn2/1 -> Product11/2, Product9/2

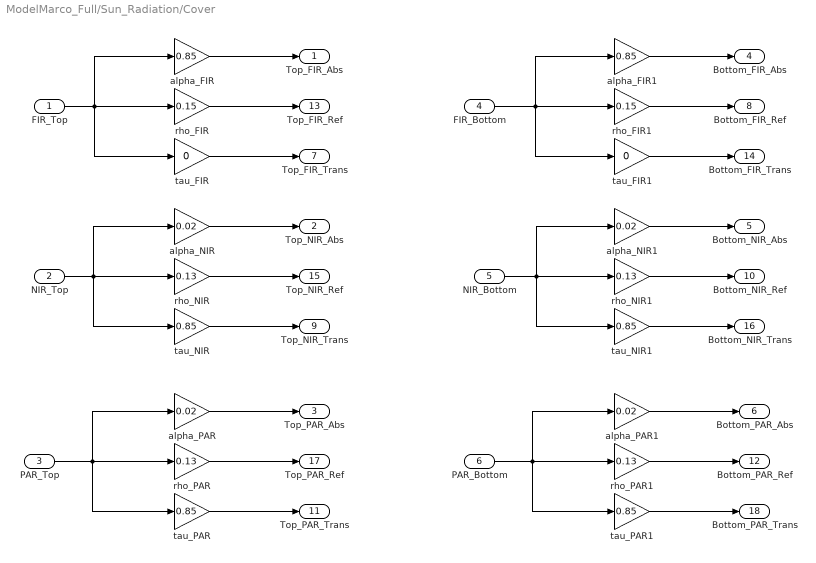
== system ModelMarco_Full/Sun_Radiation/Cover ==
  FIR_Top : Inport
  NIR_Top : Inport  Port=2
  PAR_Top : Inport  Port=3
  FIR_Bottom : Inport  Port=4
  NIR_Bottom : Inport  Port=5
  PAR_Bottom : Inport  Port=6
  alpha_FIR : Gain  Gain=0.85
  alpha_FIR1 : Gain  Gain=0.85
  alpha_NIR : Gain  Gain=0.02
  alpha_NIR1 : Gain  Gain=0.02
  alpha_PAR : Gain  Gain=0.02
  alpha_PAR1 : Gain  Gain=0.02
  rho_FIR : Gain  Gain=0.15
  rho_FIR1 : Gain  Gain=0.15
  rho_NIR : Gain  Gain=0.13
  rho_NIR1 : Gain  Gain=0.13
  rho_PAR : Gain  Gain=0.13
  rho_PAR1 : Gain  Gain=0.13
  tau_FIR : Gain  Gain=0
  tau_FIR1 : Gain  Gain=0
  tau_NIR : Gain  Gain=0.85
  tau_NIR1 : Gain  Gain=0.85
  tau_PAR : Gain  Gain=0.85
  tau_PAR1 : Gain  Gain=0.85
  Top_FIR_Abs : Outport
  Top_NIR_Abs : Outport  Port=2
  Top_PAR_Abs : Outport  Port=3
  Bottom_FIR_Abs : Outport  Port=4
  Bottom_NIR_Abs : Outport  Port=5
  Bottom_PAR_Abs : Outport  Port=6
  Top_FIR_Trans : Outport  Port=7
  Bottom_FIR_Ref : Outport  Port=8
  Top_NIR_Trans : Outport  Port=9
  Bottom_NIR_Ref : Outport  Port=10
  Top_PAR_Trans : Outport  Port=11
  Bottom_PAR_Ref : Outport  Port=12
  Top_FIR_Ref : Outport  Port=13
  Bottom_FIR_Trans : Outport  Port=14
  Top_NIR_Ref : Outport  Port=15
  Bottom_NIR_Trans : Outport  Port=16
  Top_PAR_Ref : Outport  Port=17
  Bottom_PAR_Trans : Outport  Port=18
  wires:
  tau_FIR/1 -> Top_FIR_Trans/1
  rho_FIR/1 -> Top_FIR_Ref/1
  FIR_Top/1 -> tau_FIR/1, alpha_FIR/1, rho_FIR/1
  alpha_FIR/1 -> Top_FIR_Abs/1
  FIR_Bottom/1 -> tau_FIR1/1, alpha_FIR1/1, rho_FIR1/1
  rho_FIR1/1 -> Bottom_FIR_Ref/1
  tau_FIR1/1 -> Bottom_FIR_Trans/1
  alpha_FIR1/1 -> Bottom_FIR_Abs/1
  rho_NIR/1 -> Top_NIR_Ref/1
  tau_NIR/1 -> Top_NIR_Trans/1
  NIR_Top/1 -> tau_NIR/1, rho_NIR/1, alpha_NIR/1
  alpha_NIR/1 -> Top_NIR_Abs/1
  rho_NIR1/1 -> Bottom_NIR_Ref/1
  NIR_Bottom/1 -> alpha_NIR1/1, rho_NIR1/1, tau_NIR1/1
  alpha_NIR1/1 -> Bottom_NIR_Abs/1
  tau_NIR1/1 -> Bottom_NIR_Trans/1
  tau_PAR/1 -> Top_PAR_Trans/1
  rho_PAR/1 -> Top_PAR_Ref/1
  alpha_PAR/1 -> Top_PAR_Abs/1
  PAR_Top/1 -> tau_PAR/1, alpha_PAR/1, rho_PAR/1
  tau_PAR1/1 -> Bottom_PAR_Trans/1
  rho_PAR1/1 -> Bottom_PAR_Ref/1
  alpha_PAR1/1 -> Bottom_PAR_Abs/1
  PAR_Bottom/1 -> tau_PAR1/1, alpha_PAR1/1, rho_PAR1/1

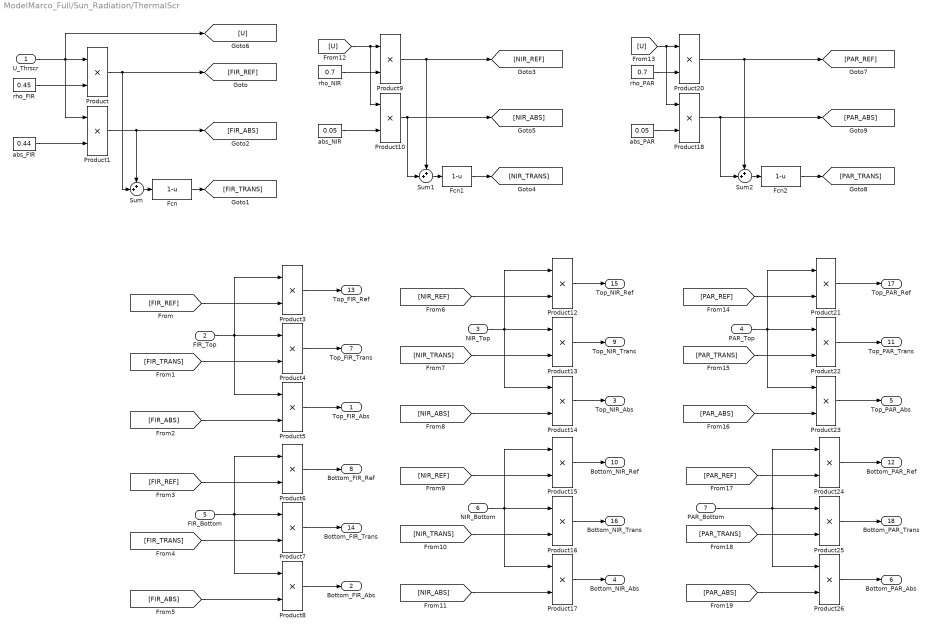
== system ModelMarco_Full/Sun_Radiation/ThermalScr ==
  U_Thrscr : Inport
  FIR_Top : Inport  Port=2
  NIR_Top : Inport  Port=3
  PAR_Top : Inport  Port=4
  FIR_Bottom : Inport  Port=5
  NIR_Bottom : Inport  Port=6
  PAR_Bottom : Inport  Port=7
  Fcn : Fcn  Expr=1-u
  Fcn1 : Fcn  Expr=1-u
  Fcn2 : Fcn  Expr=1-u
  Product{,1,3..10,12..18,20..26} (24 alike) : Product
  Sum : Sum  Inputs=++|
  Sum1 : Sum  Inputs=++|
  Sum2 : Sum  Inputs=++|
  abs_FIR : Constant  Value=0.44
  abs_NIR : Constant  Value=0.05
  abs_PAR : Constant  Value=0.05
  rho_FIR : Constant  Value=0.45
  rho_NIR : Constant  Value=0.7
  rho_PAR : Constant  Value=0.7
  Top_FIR_Abs : Outport
  Bottom_FIR_Abs : Outport  Port=2
  Top_NIR_Abs : Outport  Port=3
  Bottom_NIR_Abs : Outport  Port=4
  Top_PAR_Abs : Outport  Port=5
  Bottom_PAR_Abs : Outport  Port=6
  Top_FIR_Trans : Outport  Port=7
  Bottom_FIR_Ref : Outport  Port=8
  Top_NIR_Trans : Outport  Port=9
  Bottom_NIR_Ref : Outport  Port=10
  Top_PAR_Trans : Outport  Port=11
  Bottom_PAR_Ref : Outport  Port=12
  Top_FIR_Ref : Outport  Port=13
  Bottom_FIR_Trans : Outport  Port=14
  Top_NIR_Ref : Outport  Port=15
  Bottom_NIR_Trans : Outport  Port=16
  Top_PAR_Ref : Outport  Port=17
  Bottom_PAR_Trans : Outport  Port=18
  wires:
  FIR_Top/1 -> Product3/1, Product5/1, Product4/1
  abs_FIR/1 -> Product1/2
  U_Thrscr/1 -> Product1/1, Product/1, [U]
  Fcn/1 -> [FIR_TRANS]
  rho_FIR/1 -> Product/2
  Sum/1 -> Fcn/1
  Product/1 -> Sum/2, [FIR_REF]
  [FIR_REF] -> Product3/2
  Product4/1 -> Top_FIR_Trans/1
  Product3/1 -> Top_FIR_Ref/1
  Product6/1 -> Bottom_FIR_Ref/1
  Product7/1 -> Bottom_FIR_Trans/1
  Product5/1 -> Top_FIR_Abs/1
  Product8/1 -> Bottom_FIR_Abs/1
  [FIR_ABS] -> Product5/2
  [FIR_TRANS] -> Product4/2
  [FIR_TRANS] -> Product7/2
  [FIR_ABS] -> Product8/2
  FIR_Bottom/1 -> Product6/1, Product8/1, Product7/1
  [FIR_REF] -> Product6/2
  abs_NIR/1 -> Product10/2
  rho_NIR/1 -> Product9/2
  Sum1/1 -> Fcn1/1
  Product9/1 -> Sum1/1, [NIR_REF]
  [NIR_TRANS] -> Product13/2
  [NIR_REF] -> Product12/2
  NIR_Top/1 -> Product12/1, Product14/1, Product13/1
  [NIR_ABS] -> Product14/2
  [NIR_REF] -> Product15/2
  [NIR_ABS] -> Product17/2
  [NIR_TRANS] -> Product16/2
  NIR_Bottom/1 -> Product15/1, Product17/1, Product16/1
  Product14/1 -> Top_NIR_Abs/1
  Product13/1 -> Top_NIR_Trans/1
  Product12/1 -> Top_NIR_Ref/1
  Product15/1 -> Bottom_NIR_Ref/1
  Product16/1 -> Bottom_NIR_Trans/1
  Product17/1 -> Bottom_NIR_Abs/1
  [U] -> Product10/1, Product9/1
  [U] -> Product18/1, Product20/1
  Sum2/1 -> Fcn2/1
  rho_PAR/1 -> Product20/2
  abs_PAR/1 -> Product18/2
  [PAR_REF] -> Product21/2
  PAR_Top/1 -> Product21/1, Product23/1, Product22/1
  [PAR_TRANS] -> Product22/2
  [PAR_ABS] -> Product23/2
  Product21/1 -> Top_PAR_Ref/1
  Product22/1 -> Top_PAR_Trans/1
  Product23/1 -> Top_PAR_Abs/1
  Product26/1 -> Bottom_PAR_Abs/1
  [PAR_ABS] -> Product26/2
  [PAR_REF] -> Product24/2
  [PAR_TRANS] -> Product25/2
  Product24/1 -> Bottom_PAR_Ref/1
  Product25/1 -> Bottom_PAR_Trans/1
  PAR_Bottom/1 -> Product24/1, Product26/1, Product25/1
  Product1/1 -> Sum/1, [FIR_ABS]
  Product10/1 -> [NIR_ABS], Sum1/2
  Fcn1/1 -> [NIR_TRANS]
  Fcn2/1 -> [PAR_TRANS]
  Product18/1 -> Sum2/2, [PAR_ABS]
  Product20/1 -> Sum2/1, [PAR_REF]

== system ModelMarco_Full/Sun_Radiation/floor ==
  FIR_Top : Inport
  NIR_Top : Inport  Port=2
  PAR_Top : Inport  Port=3
  alpha_FIR : Gain
  alpha_NIR : Gain  Gain=0.5
  alpha_PAR : Gain  Gain=0.35
  rho_FIR : Gain  Gain=0
  rho_NIR : Gain  Gain=0.5
  rho_PAR : Gain  Gain=0.65
  tau_FIR : Gain  Gain=0
  tau_NIR : Gain  Gain=0
  tau_PAR : Gain  Gain=0
  Top_FIR_Abs : Outport
  Top_NIR_Abs : Outport  Port=2
  Top_PAR_Abs : Outport  Port=3
  Top_FIR_Ref : Outport  Port=4
  Top_NIR_Ref : Outport  Port=5
  Top_PAR_Ref : Outport  Port=6
  Top_FIR_Trans : Outport  Port=7
  Top_NIR_Trans : Outport  Port=8
  Top_PAR_Trans : Outport  Port=9
  wires:
  tau_FIR/1 -> Top_FIR_Trans/1
  rho_FIR/1 -> Top_FIR_Ref/1
  FIR_Top/1 -> tau_FIR/1, alpha_FIR/1, rho_FIR/1
  alpha_FIR/1 -> Top_FIR_Abs/1
  rho_NIR/1 -> Top_NIR_Ref/1
  tau_NIR/1 -> Top_NIR_Trans/1
  NIR_Top/1 -> tau_NIR/1, rho_NIR/1, alpha_NIR/1
  alpha_NIR/1 -> Top_NIR_Abs/1
  tau_PAR/1 -> Top_PAR_Trans/1
  rho_PAR/1 -> Top_PAR_Ref/1
  alpha_PAR/1 -> Top_PAR_Abs/1
  PAR_Top/1 -> tau_PAR/1, alpha_PAR/1, rho_PAR/1

== system ModelMarco_Full/Plants(transpiration)/Stomatal Resistance /CO2 plenaty factor ==
  C_CO2 : Inport
  I_d/n : Inport  Port=2
  I_A_can : Inport  Port=3
  Bias6 : Bias  Bias=-200
  Bias7 : Bias  Bias=1
  Bias8 : Bias  Bias=1
  Gain5 : Gain  Gain=6.08e-7
  Gain6 : Gain  Gain=1.1e-11
  MATLAB Function1 : MATLAB Function  TreatAsAtomicUnit=on
  MATLAB Function2 : MATLAB Function  TreatAsAtomicUnit=on
  Math Function3 : Math  Operator=magnitude^2  SaturateOnIntegerOverflow=on
  max : Constant  Value=1.49
  max_CO2 : Constant  Value=1100
  f(C_CO2) : Outport
  wires:
  Math Function3/1 -> Gain6/1, Gain5/1
  MATLAB Function1/1(Out) -> MATLAB Function2/2(u_lower)
  C_CO2/1 -> MATLAB Function2/4(key), Bias6/1
  max/1 -> MATLAB Function2/1(u_upper)
  Gain6/1 -> Bias8/1
  I_A_can/1 -> MATLAB Function1/4(key)
  Gain5/1 -> Bias7/1
  Bias8/1 -> MATLAB Function1/2(u_lower)
  max_CO2/1 -> MATLAB Function2/3(thres)
  Bias6/1 -> Math Function3/1
  Bias7/1 -> MATLAB Function1/1(u_upper)
  I_d/n/1 -> MATLAB Function1/3(thres)
  MATLAB Function2/1(Out) -> f(C_CO2)/1  "f(C_CO2)"

== system ModelMarco_Full/Plants(transpiration)/Stomatal Resistance /Radiation plenaty facor ==
  PAR : Inport
  LAI : Inport  Port=2
  Bias : Bias  Bias=4.3
  Bias1 : Bias  Bias=0.54
  Divide2 : Product  Inputs=*/
  Divide3 : Product  Inputs=*/
  Gain2 : Gain  Gain=2
  f(I_sun) : Outport
  wires:
  Bias1/1 -> Divide3/2
  Gain2/1 -> Divide2/2
  LAI/1 -> Gain2/1
  Divide2/1 -> Bias/1, Bias1/1
  Bias/1 -> Divide3/1
  Divide3/1 -> f(I_sun)/1  "f(I_sun)"
  PAR/1 -> Divide2/1

== system ModelMarco_Full/Plants(transpiration)/Stomatal Resistance /Subsystem ==
  I_d/n : Inport
  I_A_can : Inport  Port=2
  VP : Inport  Port=3
  VP_S : Inport  Port=4
  Fcn4 : Fcn  Expr=4.3e-6 * u +1
  Fcn5 : Fcn  Expr=5.2e-6 * u +1
  MATLAB Function3 : MATLAB Function  TreatAsAtomicUnit=on
  Math Function4 : Math  Operator=magnitude^2  SaturateOnIntegerOverflow=on
  Saturation : Saturate  UpperLimit=3.9
  Sum2 : Sum  Inputs=|+-
  f(C_H2O) : Outport
  wires:
  I_A_can/1 -> MATLAB Function3/4(key)
  Fcn5/1 -> MATLAB Function3/2(u_lower)
  Saturation/1 -> f(C_H2O)/1  "f(C_H2O)"
  Math Function4/1 -> Fcn5/1, Fcn4/1
  Sum2/1 -> Math Function4/1
  Fcn4/1 -> MATLAB Function3/1(u_upper)
  MATLAB Function3/1(Out) -> Saturation/1
  VP/1 -> Sum2/1
  VP_S/1 -> Sum2/2
  I_d/n/1 -> MATLAB Function3/3(thres)

== system ModelMarco_Full/Plants(transpiration)/Stomatal Resistance /Temperature Plenaty factor ==
  T_can : Inport
  I_d/n : Inport  Port=2
  I_A_can : Inport  Port=3
  Bias2 : Bias  Bias=-33.6
  Bias3 : Bias  Bias=1
  Bias4 : Bias  Bias=-24.512
  Bias5 : Bias  Bias=1
  Gain3 : Gain  Gain=0.5e-2
  Gain4 : Gain  Gain=2.2593e-2
  MATLAB Function : MATLAB Function  TreatAsAtomicUnit=on
  Math Function1 : Math  Operator=magnitude^2  SaturateOnIntegerOverflow=on
  Math Function2 : Math  Operator=magnitude^2  SaturateOnIntegerOverflow=on
  f(Tcan) : Outport
  wires:
  Bias4/1 -> Math Function2/1
  Bias2/1 -> Math Function1/1
  Gain4/1 -> Bias5/1
  Math Function1/1 -> Gain3/1
  Bias3/1 -> MATLAB Function/2(u_lower)
  T_can/1 -> Bias2/1, Bias4/1
  Math Function2/1 -> Gain4/1
  Gain3/1 -> Bias3/1
  Bias5/1 -> MATLAB Function/1(u_upper)
  I_d/n/1 -> MATLAB Function/3(thres)
  I_A_can/1 -> MATLAB Function/4(key)
  MATLAB Function/1(Out) -> f(Tcan)/1  "f(Tcan)"

== matlab function ModelMarco_Full/Plants(transpiration)/Stomatal Resistance /CO2 plenaty factor/MATLAB Function1 ==
  data: u_upper input; Out output; u_lower input; thres input; key input
function Out = Smoothing(u_upper,u_lower,thres,key)
    SFL = 1/(1 + exp( 50 * (key - thres)));
    SFH = 1/(1 + exp( -50 * (key - thres)));
    Out = u_upper * SFH + u_lower * SFL;
end

== matlab function ModelMarco_Full/Plants(transpiration)/Stomatal Resistance /Temperature Plenaty factor/MATLAB Function ==
  data: u_upper input; Out output; u_lower input; thres input; key input
function Out = Smoothing(u_upper,u_lower,thres,key)
    SFL = 1/(1 + exp( 50 * (key - thres)));
    SFH = 1/(1 + exp( -50 * (key - thres)));
    Out = u_upper * SFH + u_lower * SFL;
end

== matlab function ModelMarco_Full/Plants(transpiration)/Stomatal Resistance /CO2 plenaty factor/MATLAB Function2 ==
  data: u_upper input; Out output; u_lower input; thres input; key input
function Out = Smoothing(u_upper,u_lower,thres,key)
    SFL = 1/(1 + exp( 50 * (key - thres)));
    SFH = 1/(1 + exp( -50 * (key - thres)));
    Out = u_upper * SFH + u_lower * SFL;
end

== matlab function ModelMarco_Full/Plants(transpiration)/Stomatal Resistance /Subsystem/MATLAB Function3 ==
  data: u_upper input; Out output; u_lower input; thres input; key input
function Out = Smoothing(u_upper,u_lower,thres,key)
    SFL = 1/(1 + exp( 50 * (key - thres)));
    SFH = 1/(1 + exp( -50 * (key - thres)));
    Out = u_upper * SFH + u_lower * SFL;
end

== matlab function ModelMarco_Full/Plants(transpiration)/MATLAB Function4 ==
  data: u_upper input; Out output; u_lower input; thres input; key input
function Out = Smoothing(u_upper,u_lower,thres,key)
    SFL = 1/(1 + exp( 50 * (key - thres)));
    SFH = 1/(1 + exp( -50 * (key - thres)));
    Out = u_upper * SFH + u_lower * SFL;
    if Out < 0 
        Out = 0;
    end
end

== matlab function ModelMarco_Full/Air -> Floor/MATLAB Function2 ==
  data: u_upper input; Out output; u_lower input; thres input; key input
function Out = Smoothing(u_upper,u_lower,thres,key)
    SFL = 1/(1 + exp( 50 * (key - thres)));
    SFH = 1/(1 + exp( -50 * (key - thres)));
    Out = u_upper * SFH + u_lower * SFL;
end

== matlab function ModelMarco_Full/MATLAB Function ==
  data: Temp input; VP_sat output
function VP_sat = satVP(Temp)
    VP_h = 610.780 * exp(17.08085 * Temp/(234.175 + Temp));
    VP_l = 610.714 * exp(22.44294 * Temp/(272.440 + Temp));
    SF_H = 1/(1 + exp(-50 * Temp));
    SF_L = 1/(1 + exp(50 * Temp));
    VP_sat = VP_h * SF_H + VP_l * SF_L;
end

== matlab function ModelMarco_Full/Cover(out->covout)/MATLAB Function1 ==
  data: u_upper input; Out output; u_lower input; thres input; key input
function Out = Smoothing(u_upper,u_lower,thres,key)
    SFL = 1/(1 + exp( 50 * (key - thres)));
    SFH = 1/(1 + exp( -50 * (key - thres)));
    Out = u_upper * SFH + u_lower * SFL;
end

== matlab function ModelMarco_Full/Cover(Condensation)/MATLAB Function2 ==
  data: u_upper input; Out output; u_lower input; thres input; key input
function Out = Smoothing(u_upper,u_lower,thres,key)
    SFL = 1/(1 + exp( 500 * (key - thres)));
    SFH = 1/(1 + exp( -500 * (key - thres)));
    %Out = u_upper * SFH + u_lower * SFL;
    Out = u_upper * SFH + u_lower * SFL;
    if Out < 0 
        Out = 0;
    end
end

== matlab function ModelMarco_Full/Plants(transpiration)/MATLAB Function5 ==
  data: Temp input; VP_sat output
function VP_sat = satVP(Temp)
    VP_h = 610.780 * exp(17.08085 * Temp/(234.175 + Temp));
    VP_l = 610.714 * exp(22.44294 * Temp/(272.440 + Temp));
    SF_H = 1/(1 + exp(-50 * Temp));
    SF_L = 1/(1 + exp(50 * Temp));
    VP_sat = VP_h * SF_H + VP_l * SF_L;
end

== matlab function ModelMarco_Full/MATLAB Function1 ==
  data: Temp input; VP_sat output
function VP_sat = satVP(Temp)
    VP_h = 610.780 * exp(17.08085 * Temp/(234.175 + Temp));
    VP_l = 610.714 * exp(22.44294 * Temp/(272.440 + Temp));
    SF_H = 1/(1 + exp(-50 * Temp));
    SF_L = 1/(1 + exp(50 * Temp));
    VP_sat = VP_h * SF_H + VP_l * SF_L;
end

== matlab function ModelMarco_Full/ScrU(Condensation)/MATLAB Function2 ==
  data: u_upper input; Out output; u_lower input; thres input; key input
function Out = Smoothing(u_upper,u_lower,thres,key)
    SFL = 1/(1 + exp( 50 * (key - thres)));
    SFH = 1/(1 + exp( -50 * (key - thres)));
    %Out = u_upper * SFH + u_lower * SFL;
    Out = u_upper * SFH + u_lower * SFL;
    if Out < 0 
        Out = 0;
    end
end

== matlab function ModelMarco_Full/ScrB(Condensation)/MATLAB Function2 ==
  data: u_upper input; Out output; u_lower input; thres input; key input
function Out = Smoothing(u_upper,u_lower,thres,key)
    SFL = 1/(1 + exp( 50 * (key - thres)));
    SFH = 1/(1 + exp( -50 * (key - thres)));
    %Out = u_upper * SFH + u_lower * SFL;
    Out = u_upper * SFH + u_lower * SFL;
    if Out < 0 
        Out = 0;
    end
end

== matlab function ModelMarco_Full/RoofStrategy/MATLAB Function ==
  data: T_air input; y output; Tset input
function y = PT(T_air,Tset)
    if Tset - T_air > 5 % Closed it for heating up
        y = 0;
    else
        y =  1 - 0.2 * (Tset - T_air);
        if y > 1
            y = 1;
        end
    end
end

== matlab function ModelMarco_Full/RoofStrategy/MATLAB Function1 ==
  data: RH_air input; y output; RH_out input; RH_set input
function y = PRH(RH_air,RH_out,RH_set)
    if RH_set - RH_air > 10
        y = 0;
    else
        y = 1 - 0.1 * (RH_set - RH_air);
        if y > 1 
            y = 1;
        end
    end
    if RH_out >= RH_air
        y = 0;
    end
end
